simulink model "GMVC_pid"  (Simulink 5.0)
settings: Solver=ode45  StartTime=0.0  StopTime=500.0  RelTol=1e-3
undefined symbols (not defined in the file): A, B, L, L1, Ts, zk
settings Model: Creator=kannan  LastModifiedBy=kannan  ExtModeAutoUpdateStatusClock=off

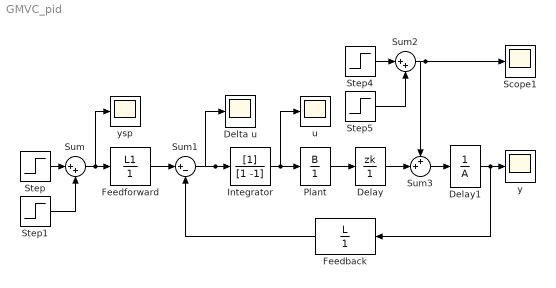
== system GMVC_pid ==
  Delay : DiscreteFilter  Numerator=zk  Denominator=1  SampleTime=Ts
  Delay1 : DiscreteFilter  Numerator=1  Denominator=A  SampleTime=Ts
  Delta u : Scope
      settings: TimeRange=500  YMin=-8  YMax=8  SaveName=ScopeData4
  Feedback : DiscreteFilter  Orientation=left  Numerator=L  Denominator=1  SampleTime=Ts
  Feedforward : DiscreteFilter  Numerator=L1  Denominator=1  SampleTime=Ts
  Integrator : DiscreteFilter  Denominator=[1 -1]
  Plant : DiscreteFilter  Numerator=B  Denominator=1  SampleTime=Ts
  Scope1 : Scope
      settings: TickLabels=on  YMin=-0.05  YMax=0.15
  Step : Step  Time=50  SampleTime=Ts
  Step1 : Step  Time=150  After=-1  SampleTime=Ts
  Step4 : Step  Time=300  After=0.1  SampleTime=Ts
  Step5 : Step  Time=400  After=-0.1  SampleTime=1
  Sum : Sum  Inputs=|++  SaturateOnIntegerOverflow=on
  Sum1 : Sum  Inputs=|+-  SaturateOnIntegerOverflow=on
  Sum2 : Sum  Inputs=|++  SaturateOnIntegerOverflow=on
  Sum3 : Sum  Inputs=++|  SaturateOnIntegerOverflow=on
  u : Scope
      settings: TimeRange=500  YMin=-2  YMax=8  SaveName=ScopeData3
  y : Scope
      settings: TimeRange=500  YMin=-0.6  YMax=1.2
  ysp : Scope
      settings: YMin=-0.2  YMax=1.2  SaveName=ScopeData2
  wires:
  Step1/1 -> Sum/2
  Step/1 -> Sum/1
  Feedforward/1 -> Sum1/1
  Step5/1 -> Sum2/2
  Step4/1 -> Sum2/1
  Feedback/1 -> Sum1/2
  Sum1/1 -> Integrator/1, Delta u/1
  Integrator/1 -> u/1, Plant/1
  Sum/1 -> Feedforward/1, ysp/1
  Sum3/1 -> Delay1/1
  Sum2/1 -> Scope1/1, Sum3/1
  Plant/1 -> Delay/1
  Delay/1 -> Sum3/2
  Delay1/1 -> Feedback/1, y/1
